simulink subsystem "ControllerBA"  (R2023b)
settings: Solver=VariableStepAuto  StartTime=0.0  StopTime=10.0  RelTol=1e-3
settings Model: Creator=juana  LastModifiedBy=juana

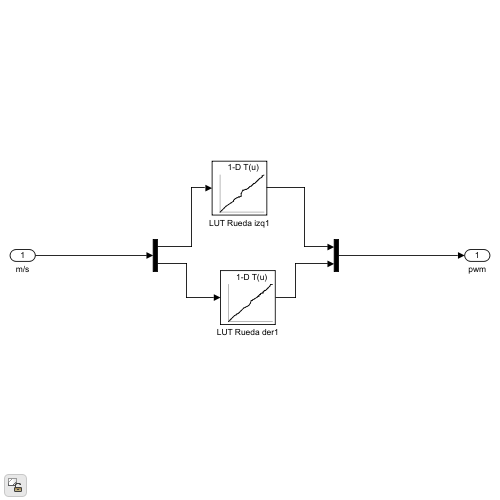
[thumbnail: Simulink's stored preview of the top-level diagram]
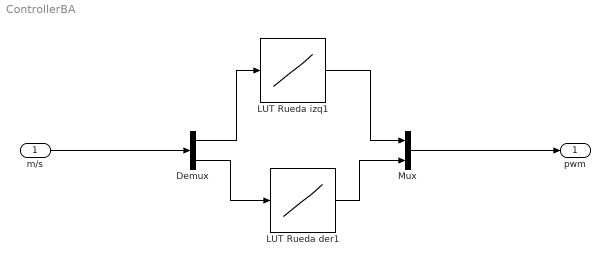
== system ControllerBA ==
  m/s : Inport
  Demux : Demux  Outputs=2
  LUT Rueda der1 : Lookup_n-D  NumberOfTableDimensions=1  BreakpointsForDimension1=[-0.880012512207031;-0.808662414550781;-0.761093139648438;-0.713516235351563;-0.642166137695313;-0.570816040039063;-0.523239135742188;-0.475677490234375;-0.4281005859375;-0.35675048828125;-0.261627197265625;-0.190277099609375;-0.1427001953125;-0.118927001953125;-0.0475616455078125;0;0.0237840451300144;0.0713521391153336;0.0951362252235413;0.166488289833069;0.261624813079834;0.285408496856689;0.309192657470703;0.332977294921875;0.35676097869873;0.380544662475586;0.404329299926758;0.42811393737793;0.475679397583008;0.499465942382813;0.523246765136719;0.547029495239258;0.594600677490234;0.618385314941406;0.642166137695313;0.689739227294922;0.713520050048828;0.784866333007813;0.832443237304688;0.8800048828125]  Table=[-254;-233.679962158203;-215.899978637695;-200.65998840332;-175.259948730469;-162.559967041016;-149.859985351563;-134.619995117188;-125.729972839355;-100.32999420166;-74.9299621582031;-58.4200057983398;-50.8000106811523;-44.4499893188477;-34.2899971008301;0;33.1499977111816;38.2499923706055;43.3499908447266;51.0000114440918;75.2249908447266;84.1499938964844;89.2499923706055;95.625;100.724998474121;108.374984741211;114.75;124.949989318848;135.150024414063;141.524993896484;150.450012207031;155.550003051758;168.299987792969;174.674987792969;182.324981689453;195.074996948242;200.175018310547;225.675003051758;244.79997253418;255]  InternalRulePriority=Speed  RndMeth=Simplest
  LUT Rueda izq1 : Lookup_n-D  NumberOfTableDimensions=1  BreakpointsForDimension1=[-0.856231689453125;-0.784873962402344;-0.689743041992188;-0.618392944335938;-0.523239135742188;-0.428115844726563;-0.332962036132813;-0.309188842773438;-0.285400390625;-0.237838745117188;-0.190277099609375;-0.118927001953125;-0.0951385498046875;-0.0237884521484375;0;0.0475680977106094;0.0951361954212189;0.14270430803299;0.190272331237793;0.237840414047241;0.261624336242676;0.285408973693848;0.309191703796387;0.332977294921875;0.38054370880127;0.404329299926758;0.451896667480469;0.475681304931641;0.499465942382813;0.523248672485352;0.547033309936523;0.570816040039063;0.594600677490234;0.618385314941406;0.665950775146484;0.689739227294922;0.713520050048828;0.784873962402344;0.80865478515625;0.832443237304688;0.880012512207031]  Table=[-254;-224.789993286133;-200.65998840332;-175.259948730469;-149.859985351563;-125.729972839355;-100.32999420166;-90.1700057983398;-83.8199768066406;-74.9299621582031;-59.6899719238281;-50.8000106811523;-44.4499893188477;-33.0199699401856;0;40.799991607666;44.6250038146973;51.0000114440918;58.6499900817871;68.8499984741211;71.3999938964844;79.0500030517578;90.5249862670898;93.0750045776367;100.724998474121;113.474998474121;124.949989318848;133.875;141.524993896484;140.249984741211;150.450012207031;158.100006103516;163.199996948242;174.674987792969;183.600006103516;192.524993896484;200.174987792969;216.75;226.949996948242;234.599990844727;255]  InternalRulePriority=Speed  RndMeth=Simplest
  Mux : Mux  Inputs=2
  pwm : Outport
  wires:
  m/s/1 -> Demux/1
  Mux/1 -> pwm/1
  Demux/1 -> LUT Rueda izq1/1
  LUT Rueda izq1/1 -> Mux/1
  Demux/2 -> LUT Rueda der1/1
  LUT Rueda der1/1 -> Mux/2
